simulink model "test_bbb"  (R2014b)
settings: Solver=FixedStepDiscrete  StartTime=0.0  StopTime=Inf  FixedStep=2e-4  RelTol=1e-3
StartFcn:
  | run runtarget
libraries: simulink x1
settings Model: SimulationMode=external  ExtModeTrigDuration=1000000  Creator=bbb  LastModifiedBy=parallels
settings SolverCC: InsertRTBMode=Always
settings OptimizationCC: OptimizeModelRefInitCode=on  LifeSpan=Inf
settings RTWCC: SystemTargetFile=ert_linux.tlc  MakeCommand="make_rtw CC=arm-linux-gnueabihf-gcc CPP=arm-linux-gnueabihf-g++ OPTS=-DWITH_HW OPTIMIZATION_FLAGS=-O3 ADDITIONAL_LDFLAGS=\"-static -static-libgcc\""  TemplateMakefile=ert_linux.tmf  Description=Linux Embedded Coder  RetainRTWFile=on  ProcessScript=ert_linux_make_rtw_hook  TargetLang=C++
settings CodeAppCC: IgnoreCustomStorageClasses=off
settings STFCustomTargetCC: ModelReferenceCompliant=off  CombineOutputUpdateFcns=on  ERTCustomFileBanners=on  SupportContinuousTime=off  SupportNonInlinedSFcns=off  MATLABClassNameForMDSCustomization=Simulink.SoftwareTarget.ERTCustomization  GRTInterface=off  SystemTargetFile=ert_linux.tlc
settings ERTTargetCC: ModelReferenceCompliant=off  ParMdlRefBuildCompliant=off  CompOptLevelCompliant=off  ConcurrentExecutionCompliant=off  ERTFirstTimeCompliant=off  ModelStepFunctionPrototypeControlCompliant=off  CPPClassGenCompliant=off  ExtMode=on  ExtModeMexArgs='192.168.7.2' 1 17725  InlinedParameterPlacement=NonHierarchical  ERTCustomFileTemplate=ert_linux_file_process.tlc

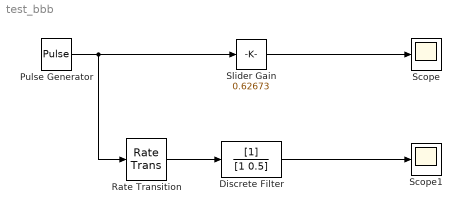
== system test_bbb ==
  Discrete Filter : DiscreteFilter
  Pulse Generator : DiscretePulseGenerator  PulseType=Time based  Amplitude=2  Period=1  PulseWidth=5
  Rate Transition : RateTransition  OutPortSampleTime=0.01
  Scope : Scope
      settings: YMin=0  YMax=3
  Scope1 : Scope
  Slider Gain : simulink/Math Operations/Slider Gain  low=0  gain=0.62673  high=2
  wires:
  Pulse Generator/1 -> Rate Transition/1, Slider Gain/1
  Rate Transition/1 -> Discrete Filter/1
  Discrete Filter/1 -> Scope1/1
  Slider Gain/1 -> Scope/1
